simulink model "switchonoff"  (Simulink 7.0)
settings: Solver=ode45  StartTime=0.0  StopTime=10.0  RelTol=1e-3
settings Model: Creator=tjjlombaerts  LastModifiedBy=tjjlombaerts

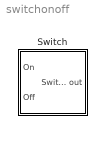
== system switchonoff ==
  Switch : Subsystem

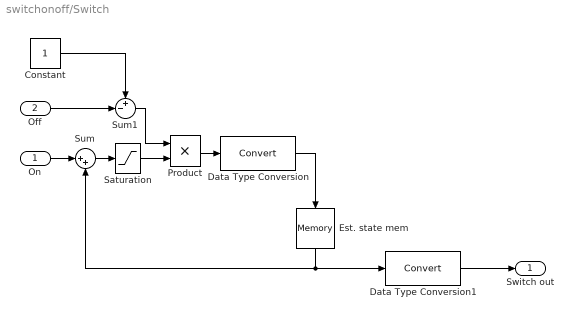
== system switchonoff/Switch ==
  On : Inport  OutDataType=sfix(16)  OutScaling=2^0
  Off : Inport  Port=2  OutDataType=sfix(16)  OutScaling=2^0
  Constant : Constant  OutDataType=sfix(16)  OutScaling=2^0
  Data Type Conversion : DataTypeConversion  OutDataTypeMode=boolean  OutDataType=sfix(16)  OutScaling=2^0
  Data Type Conversion1 : DataTypeConversion  OutDataTypeMode=double  OutDataType=sfix(16)  OutScaling=2^0
  Est. state mem : Memory  Orientation=down  InheritSampleTime=on
  Product : Product  OutDataType=sfix(16)  OutScaling=2^0  RndMeth=Zero
  Saturation : Saturate  UpperLimit=1  LowerLimit=0
  Sum : Sum  Inputs=|++  OutDataType=sfix(16)  OutScaling=2^0
  Sum1 : Sum  Inputs=+-|  OutDataType=sfix(16)  OutScaling=2^0
  Switch out : Outport  OutDataType=sfix(16)  OutScaling=2^0
  wires:
  Product/1 -> Data Type Conversion/1
  Sum/1 -> Saturation/1
  Est. state mem/1 -> Sum/2, Data Type Conversion1/1
  On/1 -> Sum/1
  Saturation/1 -> Product/2
  Sum1/1 -> Product/1
  Off/1 -> Sum1/2
  Constant/1 -> Sum1/1
  Data Type Conversion/1 -> Est. state mem/1
  Data Type Conversion1/1 -> Switch out/1
